simulink library "xrbsComm_r3"  (Simulink 5.1)
libraries: xbsIndex_r3 x775, xrbsComm_r3 x1
(part 3 of 6)

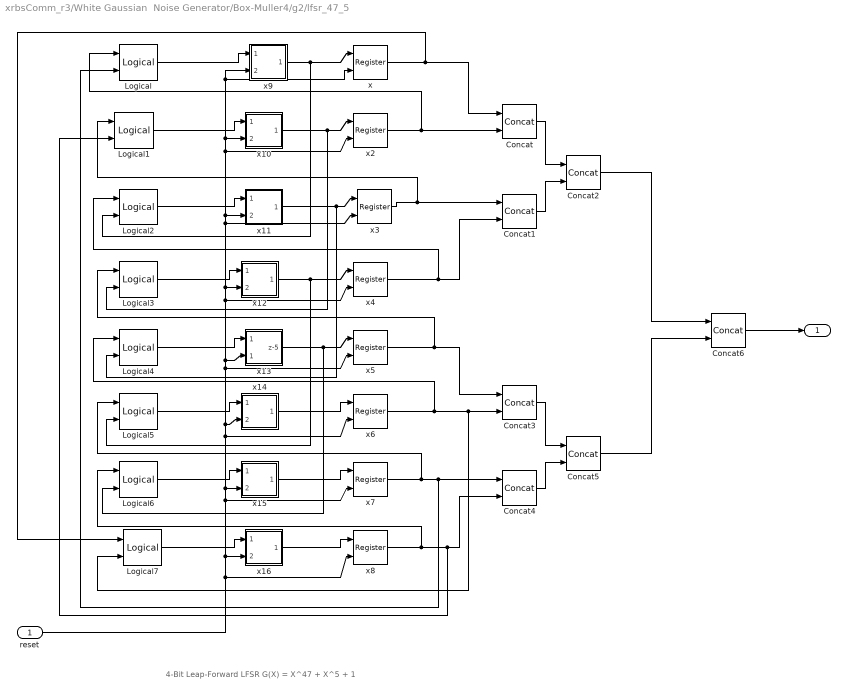
== system xrbsComm_r3/White Gaussian  Noise Generator/Box-Muller4/g2/lfsr_47_5 ==
  note: 4-Bit Leap-Forward LFSR G(X) = X^47 + X^5 + 1
  reset : Inport
  Concat{,1..6} (7 alike) : xbsIndex_r3/Concat  explicit_period=off  period=1  dbl_ovrd=off
  Logical{,1..7} (8 alike) : xbsIndex_r3/Logical  logical_function=XOR  inputs=2  precision=User Defined  arith_type=Unsigned  n_bits=1  bin_pt=0  align_bp=on  latency=0  explicit_period=on  period=-1  en=off  dbl_ovrd=off
      settings: xl_area=[0, 0, 0, 0, 0, 0, 0]
  x : xbsIndex_r3/Register  init=init(1)  reg_only_valid=off  explicit_period=off  period=1  rst=on  en=off  out_en=off  dbl_ovrd=off
      settings: xl_area=[0, 0, 0, 0, 0, 0, 0]
  x10 : Subsystem  mask{init=init(10:8:42)}
  x11 : Subsystem  mask{init=init(11:8:43)}
  x12 : Subsystem  mask{init=init(12:8:44)}
  x13 : Subsystem  mask{init=init(13:8:45)}
  x14 : Subsystem  mask{init=init(14:8:46)}
  x15 : Subsystem  mask{init=init(15:8:47)}
  x16 : Subsystem  mask{init=init(16:8:40)}
  x2 : xbsIndex_r3/Register  init=init(2)  reg_only_valid=off  explicit_period=off  period=1  rst=on  en=off  out_en=off  dbl_ovrd=off
      settings: xl_area=[0, 0, 0, 0, 0, 0, 0]
  x3 : xbsIndex_r3/Register  init=init(3)  reg_only_valid=off  explicit_period=off  period=1  rst=on  en=off  out_en=off  dbl_ovrd=off
      settings: xl_area=[0, 0, 0, 0, 0, 0, 0]
  x4 : xbsIndex_r3/Register  init=init(4)  reg_only_valid=off  explicit_period=off  period=1  rst=on  en=off  out_en=off  dbl_ovrd=off
      settings: xl_area=[0, 0, 0, 0, 0, 0, 0]
  x5 : xbsIndex_r3/Register  init=init(5)  reg_only_valid=off  explicit_period=off  period=1  rst=on  en=off  out_en=off  dbl_ovrd=off
      settings: xl_area=[0, 0, 0, 0, 0, 0, 0]
  x6 : xbsIndex_r3/Register  init=init(6)  reg_only_valid=off  explicit_period=off  period=1  rst=on  en=off  out_en=off  dbl_ovrd=off
      settings: xl_area=[0, 0, 0, 0, 0, 0, 0]
  x7 : xbsIndex_r3/Register  init=init(7)  reg_only_valid=off  explicit_period=off  period=1  rst=on  en=off  out_en=off  dbl_ovrd=off
      settings: xl_area=[0, 0, 0, 0, 0, 0, 0]
  x8 : xbsIndex_r3/Register  init=init(8)  reg_only_valid=off  explicit_period=off  period=1  rst=on  en=off  out_en=off  dbl_ovrd=off
      settings: xl_area=[0, 0, 0, 0, 0, 0, 0]
  x9 : Subsystem  mask{init=init(9:8:41)}
  " " : Outport
  wires:
  Logical/1 -> x9/1(" ")
  x9/1(z-5) -> x/1, Logical2/2
  x/1 -> Concat/1, Logical7/1
  x2/1 -> Concat/2, Logical/1
  Concat/1 -> Concat2/1
  x3/1 -> Concat1/1, Logical1/1
  x4/1 -> Concat1/2, Logical2/1
  Concat1/1 -> Concat2/2
  Logical1/1 -> x10/1("  ")
  x10/1(z-5) -> x2/1, Logical3/2
  Logical2/1 -> x11/1(" ")
  x11/1(z-5) -> x3/1, Logical4/2
  Logical3/1 -> x12/1(" ")
  x12/1(z-5) -> x4/1, Logical5/2
  Logical4/1 -> x13/1(" ")
  x13/1(z-5) -> x5/1, Logical6/2
  Logical5/1 -> x14/1(" ")
  x14/1(z-5) -> x6/1
  Logical6/1 -> x15/1(" ")
  x15/1(z-5) -> x7/1
  Logical7/1 -> x16/1(" ")
  x16/1(z-4) -> x8/1
  x6/1 -> Logical4/1, Concat3/2, Logical7/2
  Concat3/1 -> Concat5/1
  Concat4/1 -> Concat5/2
  x5/1 -> Concat3/1, Logical3/1
  x7/1 -> Concat4/1, Logical/2, Logical5/1
  x8/1 -> Concat4/2, Logical1/2, Logical6/1
  Concat2/1 -> Concat6/1
  Concat5/1 -> Concat6/2
  Concat6/1 -> " "/1
  reset/1 -> x9/2(reset), x/2, x10/2(reset), x2/2, x11/2(reset), x3/2, x12/2(reset), x4/2, x13/2(" 1"), x5/2, x14/2(reset), x6/2, x15/2(reset), x7/2, x16/2(reset), x8/2

== system xrbsComm_r3/White Gaussian  Noise Generator/Box-Muller1/f/lfsr_17_2/x1 ==
  " " : Inport
  " reset" : Inport  Port=2
  ASR : Subsystem  mask{init=[init(1) init(2)]}
      mask prompts: init "Initial Value"
      mask init:
      | init_size = size(init);
      | asr_length = init_size(2);
  Register4 : xbsIndex_r3/Register  init=init(3)  reg_only_valid=off  explicit_period=on  period=-1  rst=on  en=off  out_en=off  dbl_ovrd=off
      settings: xl_area=[0, 0, 0, 0, 0, 0, 0]
  z-3 : Outport
  wires:
  " "/1 -> Register4/1
  ASR/1(dout) -> z-3/1
  Register4/1 -> ASR/1(din)
  " reset"/1 -> Register4/2

== system xrbsComm_r3/White Gaussian  Noise Generator/Box-Muller1/f/lfsr_17_2/x5 ==
  " " : Inport
  reset : Inport  Port=2
  ASR : Subsystem  mask{init=[init(1) init(2) init(3)]}
      mask prompts: init "Initial Value"
      mask init:
      | init_size = size(init);
      | asr_length = init_size(2);
  Register5 : xbsIndex_r3/Register  init=init(4)  reg_only_valid=off  explicit_period=on  period=-1  rst=on  en=off  out_en=off  dbl_ovrd=off
      settings: xl_area=[0, 0, 0, 0, 0, 0, 0]
  z-4 : Outport
  wires:
  ASR/1(dout) -> z-4/1
  Register5/1 -> ASR/1(din)
  " "/1 -> Register5/1
  reset/1 -> Register5/2

== system xrbsComm_r3/White Gaussian  Noise Generator/Box-Muller1/f/lfsr_17_2/x6 ==
  " " : Inport
  " reset" : Inport  Port=2
  ASR : Subsystem  mask{init=[init(2) init(1)]}
      mask prompts: init "Initial Value"
      mask init:
      | init_size = size(init);
      | asr_length = init_size(2);
  Register4 : xbsIndex_r3/Register  init=init(3)  reg_only_valid=off  explicit_period=on  period=-1  rst=on  en=off  out_en=off  dbl_ovrd=off
      settings: xl_area=[0, 0, 0, 0, 0, 0, 0]
  z-3 : Outport
  wires:
  ASR/1(dout) -> z-3/1
  " "/1 -> Register4/1
  Register4/1 -> ASR/1(din)
  " reset"/1 -> Register4/2

== system xrbsComm_r3/White Gaussian  Noise Generator/Box-Muller1/f/lfsr_17_2/x7 ==
  " " : Inport
  reset : Inport  Port=2
  ASR : Subsystem  mask{init=[init(2) init(1)]}
      mask prompts: init "Initial Value"
      mask init:
      | init_size = size(init);
      | asr_length = init_size(2);
  Register4 : xbsIndex_r3/Register  init=init(3)  reg_only_valid=off  explicit_period=on  period=-1  rst=on  en=off  out_en=off  dbl_ovrd=off
      settings: xl_area=[0, 0, 0, 0, 0, 0, 0]
  z-3 : Outport
  wires:
  " "/1 -> Register4/1
  ASR/1(dout) -> z-3/1
  Register4/1 -> ASR/1(din)
  reset/1 -> Register4/2

== system xrbsComm_r3/White Gaussian  Noise Generator/Box-Muller1/f/lfsr_25_1/x1 ==
  " " : Inport
  reset : Inport  Port=2
  ASR : Subsystem  mask{init=[init(4) init(3) init(2) init(1)]}
      mask prompts: init "Initial Value"
      mask init:
      | init_size = size(init);
      | asr_length = init_size(2);
  Register : xbsIndex_r3/Register  init=init(5)  reg_only_valid=off  explicit_period=on  period=-1  rst=on  en=off  out_en=off  dbl_ovrd=off
      settings: xl_area=[0, 0, 0, 0, 0, 0, 0]
  z-5 : Outport
  wires:
  Register/1 -> ASR/1(din)
  ASR/1(dout) -> z-5/1
  " "/1 -> Register/1
  reset/1 -> Register/2

== system xrbsComm_r3/White Gaussian  Noise Generator/Box-Muller1/f/lfsr_25_1/x5 ==
  " " : Inport
  reset : Inport  Port=2
  ASR : Subsystem  mask{init=[init(5) init(4) init(3) init(2) init(1)]}
      mask prompts: init "Initial Value"
      mask init:
      | init_size = size(init);
      | asr_length = init_size(2);
  Register : xbsIndex_r3/Register  init=init(6)  reg_only_valid=off  explicit_period=on  period=-1  rst=on  en=off  out_en=off  dbl_ovrd=off
      settings: xl_area=[0, 0, 0, 0, 0, 0, 0]
  z-6 : Outport
  wires:
  Register/1 -> ASR/1(din)
  ASR/1(dout) -> z-6/1
  " "/1 -> Register/1
  reset/1 -> Register/2

== system xrbsComm_r3/White Gaussian  Noise Generator/Box-Muller1/f/lfsr_25_1/x6 ==
  " " : Inport
  reset : Inport  Port=2
  ASR : Subsystem  mask{init=[init(4) init(3) init(2) init(1)]}
      mask prompts: init "Initial Value"
      mask init:
      | init_size = size(init);
      | asr_length = init_size(2);
  Register : xbsIndex_r3/Register  init=init(5)  reg_only_valid=off  explicit_period=on  period=-1  rst=on  en=off  out_en=off  dbl_ovrd=off
      settings: xl_area=[0, 0, 0, 0, 0, 0, 0]
  z-5 : Outport
  wires:
  Register/1 -> ASR/1(din)
  ASR/1(dout) -> z-5/1
  " "/1 -> Register/1
  reset/1 -> Register/2

== system xrbsComm_r3/White Gaussian  Noise Generator/Box-Muller1/f/lfsr_25_1/x7 ==
  " " : Inport
  reset : Inport  Port=2
  ASR : Subsystem  mask{init=[init(4) init(3) init(2) init(1)]}
      mask prompts: init "Initial Value"
      mask init:
      | init_size = size(init);
      | asr_length = init_size(2);
  Register : xbsIndex_r3/Register  init=init(5)  reg_only_valid=off  explicit_period=on  period=-1  rst=on  en=off  out_en=off  dbl_ovrd=off
      settings: xl_area=[0, 0, 0, 0, 0, 0, 0]
  z-5 : Outport
  wires:
  Register/1 -> ASR/1(din)
  ASR/1(dout) -> z-5/1
  " "/1 -> Register/1
  reset/1 -> Register/2

== system xrbsComm_r3/White Gaussian  Noise Generator/Box-Muller1/f/lfsr_29_2/x5 ==
  " " : Inport
  reset : Inport  Port=2
  ASR : Subsystem  mask{init=[init(6) init(5) init(4) init(3) init(2) init(1)]}
      mask prompts: init "Initial Value"
      mask init:
      | init_size = size(init);
      | asr_length = init_size(2);
  Register : xbsIndex_r3/Register  init=init(7)  reg_only_valid=off  explicit_period=on  period=-1  rst=on  en=off  out_en=off  dbl_ovrd=off
      settings: xl_area=[0, 0, 0, 0, 0, 0, 0]
  z-7 : Outport
  wires:
  ASR/1(dout) -> z-7/1
  Register/1 -> ASR/1(din)
  " "/1 -> Register/1
  reset/1 -> Register/2

== system xrbsComm_r3/White Gaussian  Noise Generator/Box-Muller1/f/lfsr_29_2/x6 ==
  " " : Inport
  reset : Inport  Port=2
  ASR : Subsystem  mask{init=[init(5) init(4) init(3) init(2) init(1)]}
      mask prompts: init "Initial Value"
      mask init:
      | init_size = size(init);
      | asr_length = init_size(2);
  Register : xbsIndex_r3/Register  init=init(6)  reg_only_valid=off  explicit_period=on  period=-1  rst=on  en=off  out_en=off  dbl_ovrd=off
      settings: xl_area=[0, 0, 0, 0, 0, 0, 0]
  z-6 : Outport
  wires:
  ASR/1(dout) -> z-6/1
  Register/1 -> ASR/1(din)
  " "/1 -> Register/1
  reset/1 -> Register/2

== system xrbsComm_r3/White Gaussian  Noise Generator/Box-Muller1/f/lfsr_29_2/x7 ==
  " " : Inport
  reset : Inport  Port=2
  ASR : Subsystem  mask{init=[init(5) init(4) init(3) init(2) init(1)]}
      mask prompts: init "Initial Value"
      mask init:
      | init_size = size(init);
      | asr_length = init_size(2);
  Register : xbsIndex_r3/Register  init=init(6)  reg_only_valid=off  explicit_period=on  period=-1  rst=on  en=off  out_en=off  dbl_ovrd=off
      settings: xl_area=[0, 0, 0, 0, 0, 0, 0]
  z-6 : Outport
  wires:
  ASR/1(dout) -> z-6/1
  Register/1 -> ASR/1(din)
  " "/1 -> Register/1
  reset/1 -> Register/2

== system xrbsComm_r3/White Gaussian  Noise Generator/Box-Muller1/f/lfsr_29_2/x8 ==
  " " : Inport
  reset : Inport  Port=2
  ASR : Subsystem  mask{init=[init(5) init(4) init(3) init(2) init(1)]}
      mask prompts: init "Initial Value"
      mask init:
      | init_size = size(init);
      | asr_length = init_size(2);
  Register : xbsIndex_r3/Register  init=init(6)  reg_only_valid=off  explicit_period=on  period=-1  rst=on  en=off  out_en=off  dbl_ovrd=off
      settings: xl_area=[0, 0, 0, 0, 0, 0, 0]
  z-6 : Outport
  wires:
  ASR/1(dout) -> z-6/1
  Register/1 -> ASR/1(din)
  " "/1 -> Register/1
  reset/1 -> Register/2

== system xrbsComm_r3/White Gaussian  Noise Generator/Box-Muller1/f/lfsr_31_2/x5 ==
  " " : Inport
  reset : Inport  Port=2
  ASR : Subsystem  mask{init=[init(6) init(5) init(4) init(3) init(2) init(1)]}
      mask prompts: init "Initial Value"
      mask init:
      | init_size = size(init);
      | asr_length = init_size(2);
  Register : xbsIndex_r3/Register  init=init(7)  reg_only_valid=off  explicit_period=on  period=-1  rst=on  en=off  out_en=off  dbl_ovrd=off
      settings: xl_area=[0, 0, 0, 0, 0, 0, 0]
  z-7 : Outport
  wires:
  Register/1 -> ASR/1(din)
  ASR/1(dout) -> z-7/1
  " "/1 -> Register/1
  reset/1 -> Register/2

== system xrbsComm_r3/White Gaussian  Noise Generator/Box-Muller1/f/lfsr_31_2/x6 ==
  " " : Inport
  reset : Inport  Port=2
  ASR : Subsystem  mask{init=[init(6) init(5) init(4) init(3) init(2) init(1)]}
      mask prompts: init "Initial Value"
      mask init:
      | init_size = size(init);
      | asr_length = init_size(2);
  Register : xbsIndex_r3/Register  init=init(7)  reg_only_valid=off  explicit_period=on  period=-1  rst=on  en=off  out_en=off  dbl_ovrd=off
      settings: xl_area=[0, 0, 0, 0, 0, 0, 0]
  z-7 : Outport
  wires:
  Register/1 -> ASR/1(din)
  " "/1 -> Register/1
  ASR/1(dout) -> z-7/1
  reset/1 -> Register/2

== system xrbsComm_r3/White Gaussian  Noise Generator/Box-Muller1/f/lfsr_31_2/x7 ==
  " " : Inport
  reset : Inport  Port=2
  ASR : Subsystem  mask{init=[init(6) init(5) init(4) init(3) init(2) init(1)]}
      mask prompts: init "Initial Value"
      mask init:
      | init_size = size(init);
      | asr_length = init_size(2);
  Register : xbsIndex_r3/Register  init=init(7)  reg_only_valid=off  explicit_period=on  period=-1  rst=on  en=off  out_en=off  dbl_ovrd=off
      settings: xl_area=[0, 0, 0, 0, 0, 0, 0]
  z-7 : Outport
  wires:
  Register/1 -> ASR/1(din)
  ASR/1(dout) -> z-7/1
  " "/1 -> Register/1
  reset/1 -> Register/2

== system xrbsComm_r3/White Gaussian  Noise Generator/Box-Muller1/f/lfsr_31_2/x8 ==
  " " : Inport
  reset : Inport  Port=2
  ASR : Subsystem  mask{init=[init(5) init(4) init(3) init(2) init(1)]}
      mask prompts: init "Initial Value"
      mask init:
      | init_size = size(init);
      | asr_length = init_size(2);
  Register : xbsIndex_r3/Register  init=init(6)  reg_only_valid=off  explicit_period=on  period=-1  rst=on  en=off  out_en=off  dbl_ovrd=off
      settings: xl_area=[0, 0, 0, 0, 0, 0, 0]
  z-6 : Outport
  wires:
  Register/1 -> ASR/1(din)
  " "/1 -> Register/1
  ASR/1(dout) -> z-6/1
  reset/1 -> Register/2

== system xrbsComm_r3/White Gaussian  Noise Generator/Box-Muller1/f/lfsr_41_2/x1 ==
  " " : Inport
  reset : Inport  Port=2
  ASR : Subsystem  mask{init=[init(8) init(7) init(6) init(5) init(4) init(3) init(2) init(1)]}
      mask prompts: init "Initial Value"
      mask init:
      | init_size = size(init);
      | asr_length = init_size(2);
  Register1 : xbsIndex_r3/Register  init=init(9)  reg_only_valid=off  explicit_period=on  period=-1  rst=on  en=off  out_en=off  dbl_ovrd=off
      settings: xl_area=[0, 0, 0, 0, 0, 0, 0]
  z-9 : Outport
  wires:
  ASR/1(dout) -> z-9/1
  " "/1 -> Register1/1
  Register1/1 -> ASR/1(din)
  reset/1 -> Register1/2

== system xrbsComm_r3/White Gaussian  Noise Generator/Box-Muller1/f/lfsr_41_2/x5 ==
  " " : Inport
  reset : Inport  Port=2
  ASR : Subsystem  mask{init=[init(9) init(8) init(7) init(6) init(5) init(4) init(3) init(2) init(1)]}
      mask prompts: init "Initial Value"
      mask init:
      | init_size = size(init);
      | asr_length = init_size(2);
  Register : xbsIndex_r3/Register  init=init(10)  reg_only_valid=off  explicit_period=on  period=-1  rst=on  en=off  out_en=off  dbl_ovrd=off
      settings: xl_area=[0, 0, 0, 0, 0, 0, 0]
  z-10 : Outport
  wires:
  Register/1 -> ASR/1(din)
  ASR/1(dout) -> z-10/1
  " "/1 -> Register/1
  reset/1 -> Register/2

== system xrbsComm_r3/White Gaussian  Noise Generator/Box-Muller1/f/lfsr_41_2/x6 ==
  " " : Inport
  reset : Inport  Port=2
  ASR : Subsystem  mask{init=[init(8) init(7) init(6) init(5) init(4) init(3) init(2) init(1)]}
      mask prompts: init "Initial Value"
      mask init:
      | init_size = size(init);
      | asr_length = init_size(2);
  Register1 : xbsIndex_r3/Register  init=init(9)  reg_only_valid=off  explicit_period=on  period=-1  rst=on  en=off  out_en=off  dbl_ovrd=off
      settings: xl_area=[0, 0, 0, 0, 0, 0, 0]
  z-9 : Outport
  wires:
  ASR/1(dout) -> z-9/1
  " "/1 -> Register1/1
  Register1/1 -> ASR/1(din)
  reset/1 -> Register1/2

== system xrbsComm_r3/White Gaussian  Noise Generator/Box-Muller1/f/lfsr_41_2/x7 ==
  " " : Inport
  reset : Inport  Port=2
  ASR : Subsystem  mask{init=[init(8) init(7) init(6) init(5) init(4) init(3) init(2) init(1)]}
      mask prompts: init "Initial Value"
      mask init:
      | init_size = size(init);
      | asr_length = init_size(2);
  Register1 : xbsIndex_r3/Register  init=init(9)  reg_only_valid=off  explicit_period=on  period=-1  rst=on  en=off  out_en=off  dbl_ovrd=off
      settings: xl_area=[0, 0, 0, 0, 0, 0, 0]
  z-9 : Outport
  wires:
  ASR/1(dout) -> z-9/1
  Register1/1 -> ASR/1(din)
  " "/1 -> Register1/1
  reset/1 -> Register1/2

== system xrbsComm_r3/White Gaussian  Noise Generator/Box-Muller1/g/lfsr_47_5/x10 ==
  "  " : Inport
  reset : Inport  Port=2
  ASR : Subsystem  mask{init=[init(4) init(3) init(2) init(1)]}
      mask prompts: init "Initial Value"
      mask init:
      | init_size = size(init);
      | asr_length = init_size(2);
  Register5 : xbsIndex_r3/Register  init=init(5)  reg_only_valid=off  explicit_period=on  period=-1  rst=on  en=off  out_en=off  dbl_ovrd=off
      settings: xl_area=[0, 0, 0, 0, 0, 0, 0]
  z-5 : Outport
  wires:
  ASR/1(dout) -> z-5/1
  Register5/1 -> ASR/1(din)
  "  "/1 -> Register5/1
  reset/1 -> Register5/2

== system xrbsComm_r3/White Gaussian  Noise Generator/Box-Muller1/g/lfsr_47_5/x11 ==
  " " : Inport
  reset : Inport  Port=2
  ASR : Subsystem  mask{init=[init(4) init(3) init(2) init(1)]}
      mask prompts: init "Initial Value"
      mask init:
      | init_size = size(init);
      | asr_length = init_size(2);
  Register : xbsIndex_r3/Register  init=init(5)  reg_only_valid=off  explicit_period=on  period=-1  rst=on  en=off  out_en=off  dbl_ovrd=off
      settings: xl_area=[0, 0, 0, 0, 0, 0, 0]
  z-5 : Outport
  wires:
  ASR/1(dout) -> z-5/1
  Register/1 -> ASR/1(din)
  " "/1 -> Register/1
  reset/1 -> Register/2

== system xrbsComm_r3/White Gaussian  Noise Generator/Box-Muller1/g/lfsr_47_5/x12 ==
  " " : Inport
  reset : Inport  Port=2
  ASR : Subsystem  mask{init=[init(4) init(3) init(2) init(1)]}
      mask prompts: init "Initial Value"
      mask init:
      | init_size = size(init);
      | asr_length = init_size(2);
  Register : xbsIndex_r3/Register  init=init(5)  reg_only_valid=off  explicit_period=on  period=-1  rst=on  en=off  out_en=off  dbl_ovrd=off
      settings: xl_area=[0, 0, 0, 0, 0, 0, 0]
  z-5 : Outport
  wires:
  ASR/1(dout) -> z-5/1
  Register/1 -> ASR/1(din)
  " "/1 -> Register/1
  reset/1 -> Register/2

== system xrbsComm_r3/White Gaussian  Noise Generator/Box-Muller1/g/lfsr_47_5/x13 ==
  note: reset
  " " : Inport
  " 1" : Inport  Port=2
  ASR : Subsystem  mask{init=[init(4) init(3) init(2) init(1)]}
      mask prompts: init "Initial Value"
      mask init:
      | init_size = size(init);
      | asr_length = init_size(2);
  Register : xbsIndex_r3/Register  init=init(5)  reg_only_valid=off  explicit_period=on  period=-1  rst=on  en=off  out_en=off  dbl_ovrd=off
      settings: xl_area=[0, 0, 0, 0, 0, 0, 0]
  z-5 : Outport
  wires:
  ASR/1(dout) -> z-5/1
  Register/1 -> ASR/1(din)
  " "/1 -> Register/1
  " 1"/1 -> Register/2

== system xrbsComm_r3/White Gaussian  Noise Generator/Box-Muller1/g/lfsr_47_5/x14 ==
  " " : Inport
  reset : Inport  Port=2
  ASR : Subsystem  mask{init=[init(4) init(3) init(2) init(1)]}
      mask prompts: init "Initial Value"
      mask init:
      | init_size = size(init);
      | asr_length = init_size(2);
  Register : xbsIndex_r3/Register  init=init(5)  reg_only_valid=off  explicit_period=on  period=-1  rst=on  en=off  out_en=off  dbl_ovrd=off
      settings: xl_area=[0, 0, 0, 0, 0, 0, 0]
  z-5 : Outport
  wires:
  ASR/1(dout) -> z-5/1
  Register/1 -> ASR/1(din)
  " "/1 -> Register/1
  reset/1 -> Register/2

== system xrbsComm_r3/White Gaussian  Noise Generator/Box-Muller1/g/lfsr_47_5/x15 ==
  " " : Inport
  reset : Inport  Port=2
  ASR : Subsystem  mask{init=[init(4) init(3) init(2) init(1)]}
      mask prompts: init "Initial Value"
      mask init:
      | init_size = size(init);
      | asr_length = init_size(2);
  Register : xbsIndex_r3/Register  init=init(5)  reg_only_valid=off  explicit_period=on  period=-1  rst=on  en=off  out_en=off  dbl_ovrd=off
      settings: xl_area=[0, 0, 0, 0, 0, 0, 0]
  z-5 : Outport
  wires:
  ASR/1(dout) -> z-5/1
  Register/1 -> ASR/1(din)
  " "/1 -> Register/1
  reset/1 -> Register/2

== system xrbsComm_r3/White Gaussian  Noise Generator/Box-Muller1/g/lfsr_47_5/x16 ==
  " " : Inport
  reset : Inport  Port=2
  ASR : Subsystem  mask{init=[init(3) init(2) init(1)]}
      mask prompts: init "Initial Value"
      mask init:
      | init_size = size(init);
      | asr_length = init_size(2);
  Register : xbsIndex_r3/Register  init=init(4)  reg_only_valid=off  explicit_period=on  period=-1  rst=on  en=off  out_en=off  dbl_ovrd=off
      settings: xl_area=[0, 0, 0, 0, 0, 0, 0]
  z-4 : Outport
  wires:
  ASR/1(dout) -> z-4/1
  Register/1 -> ASR/1(din)
  " "/1 -> Register/1
  reset/1 -> Register/2

== system xrbsComm_r3/White Gaussian  Noise Generator/Box-Muller1/g/lfsr_47_5/x9 ==
  " " : Inport
  reset : Inport  Port=2
  ASR : Subsystem  mask{init=[init(4) init(3) init(2) init(1)]}
      mask prompts: init "Initial Value"
      mask init:
      | init_size = size(init);
      | asr_length = init_size(2);
  Register : xbsIndex_r3/Register  init=init(5)  reg_only_valid=off  explicit_period=on  period=-1  rst=on  en=off  out_en=off  dbl_ovrd=off
      settings: xl_area=[0, 0, 0, 0, 0, 0, 0]
  z-5 : Outport
  wires:
  ASR/1(dout) -> z-5/1
  Register/1 -> ASR/1(din)
  " "/1 -> Register/1
  reset/1 -> Register/2

== system xrbsComm_r3/White Gaussian  Noise Generator/Box-Muller2/fr1/lfsr_17_2/x1 ==
  " " : Inport
  " reset" : Inport  Port=2
  ASR : Subsystem  mask{init=[init(2) init(1)]}
      mask prompts: init "Initial Value"
      mask init:
      | init_size = size(init);
      | asr_length = init_size(2);
  Register4 : xbsIndex_r3/Register  init=init(3)  reg_only_valid=off  explicit_period=on  period=-1  rst=on  en=off  out_en=off  dbl_ovrd=off
      settings: xl_area=[0, 0, 0, 0, 0, 0, 0]
  z-3 : Outport
  wires:
  " "/1 -> Register4/1
  ASR/1(dout) -> z-3/1
  Register4/1 -> ASR/1(din)
  " reset"/1 -> Register4/2

== system xrbsComm_r3/White Gaussian  Noise Generator/Box-Muller2/fr1/lfsr_17_2/x5 ==
  " " : Inport
  reset : Inport  Port=2
  ASR : Subsystem  mask{init=[init(3) init(2) init(1)]}
      mask prompts: init "Initial Value"
      mask init:
      | init_size = size(init);
      | asr_length = init_size(2);
  Register5 : xbsIndex_r3/Register  init=init(4)  reg_only_valid=off  explicit_period=on  period=-1  rst=on  en=off  out_en=off  dbl_ovrd=off
      settings: xl_area=[0, 0, 0, 0, 0, 0, 0]
  z-4 : Outport
  wires:
  ASR/1(dout) -> z-4/1
  Register5/1 -> ASR/1(din)
  " "/1 -> Register5/1
  reset/1 -> Register5/2

== system xrbsComm_r3/White Gaussian  Noise Generator/Box-Muller2/fr1/lfsr_17_2/x6 ==
  " " : Inport
  " reset" : Inport  Port=2
  ASR : Subsystem  mask{init=[init(2) init(1)]}
      mask prompts: init "Initial Value"
      mask init:
      | init_size = size(init);
      | asr_length = init_size(2);
  Register4 : xbsIndex_r3/Register  init=init(3)  reg_only_valid=off  explicit_period=on  period=-1  rst=on  en=off  out_en=off  dbl_ovrd=off
      settings: xl_area=[0, 0, 0, 0, 0, 0, 0]
  z-3 : Outport
  wires:
  ASR/1(dout) -> z-3/1
  " "/1 -> Register4/1
  Register4/1 -> ASR/1(din)
  " reset"/1 -> Register4/2

== system xrbsComm_r3/White Gaussian  Noise Generator/Box-Muller2/fr1/lfsr_17_2/x7 ==
  " " : Inport
  reset : Inport  Port=2
  ASR : Subsystem  mask{init=[init(2) init(1)]}
      mask prompts: init "Initial Value"
      mask init:
      | init_size = size(init);
      | asr_length = init_size(2);
  Register4 : xbsIndex_r3/Register  init=init(3)  reg_only_valid=off  explicit_period=on  period=-1  rst=on  en=off  out_en=off  dbl_ovrd=off
      settings: xl_area=[0, 0, 0, 0, 0, 0, 0]
  z-3 : Outport
  wires:
  " "/1 -> Register4/1
  ASR/1(dout) -> z-3/1
  Register4/1 -> ASR/1(din)
  reset/1 -> Register4/2

== system xrbsComm_r3/White Gaussian  Noise Generator/Box-Muller2/fr1/lfsr_25_2/x1 ==
  " " : Inport
  reset : Inport  Port=2
  ASR : Subsystem  mask{init=[init(4) init(3) init(2) init(1)]}
      mask prompts: init "Initial Value"
      mask init:
      | init_size = size(init);
      | asr_length = init_size(2);
  Register : xbsIndex_r3/Register  init=init(5)  reg_only_valid=off  explicit_period=on  period=-1  rst=on  en=off  out_en=off  dbl_ovrd=off
      settings: xl_area=[0, 0, 0, 0, 0, 0, 0]
  z-5 : Outport
  wires:
  Register/1 -> ASR/1(din)
  ASR/1(dout) -> z-5/1
  " "/1 -> Register/1
  reset/1 -> Register/2

== system xrbsComm_r3/White Gaussian  Noise Generator/Box-Muller2/fr1/lfsr_25_2/x5 ==
  " " : Inport
  reset : Inport  Port=2
  ASR : Subsystem  mask{init=[init(5) init(4) init(3) init(2) init(1)]}
      mask prompts: init "Initial Value"
      mask init:
      | init_size = size(init);
      | asr_length = init_size(2);
  Register : xbsIndex_r3/Register  init=init(6)  reg_only_valid=off  explicit_period=on  period=-1  rst=on  en=off  out_en=off  dbl_ovrd=off
      settings: xl_area=[0, 0, 0, 0, 0, 0, 0]
  z-6 : Outport
  wires:
  Register/1 -> ASR/1(din)
  ASR/1(dout) -> z-6/1
  " "/1 -> Register/1
  reset/1 -> Register/2

== system xrbsComm_r3/White Gaussian  Noise Generator/Box-Muller2/fr1/lfsr_25_2/x6 ==
  " " : Inport
  reset : Inport  Port=2
  ASR : Subsystem  mask{init=[init(4) init(3) init(2) init(1)]}
      mask prompts: init "Initial Value"
      mask init:
      | init_size = size(init);
      | asr_length = init_size(2);
  Register : xbsIndex_r3/Register  init=init(5)  reg_only_valid=off  explicit_period=on  period=-1  rst=on  en=off  out_en=off  dbl_ovrd=off
      settings: xl_area=[0, 0, 0, 0, 0, 0, 0]
  z-5 : Outport
  wires:
  Register/1 -> ASR/1(din)
  ASR/1(dout) -> z-5/1
  " "/1 -> Register/1
  reset/1 -> Register/2

== system xrbsComm_r3/White Gaussian  Noise Generator/Box-Muller2/fr1/lfsr_25_2/x7 ==
  " " : Inport
  reset : Inport  Port=2
  ASR : Subsystem  mask{init=[init(4) init(3) init(2) init(1)]}
      mask prompts: init "Initial Value"
      mask init:
      | init_size = size(init);
      | asr_length = init_size(2);
  Register : xbsIndex_r3/Register  init=init(5)  reg_only_valid=off  explicit_period=on  period=-1  rst=on  en=off  out_en=off  dbl_ovrd=off
      settings: xl_area=[0, 0, 0, 0, 0, 0, 0]
  z-5 : Outport
  wires:
  Register/1 -> ASR/1(din)
  ASR/1(dout) -> z-5/1
  " "/1 -> Register/1
  reset/1 -> Register/2

== system xrbsComm_r3/White Gaussian  Noise Generator/Box-Muller2/fr1/lfsr_29_2/x5 ==
  " " : Inport
  reset : Inport  Port=2
  ASR : Subsystem  mask{init=[init(6) init(5) init(4) init(3) init(2) init(1)]}
      mask prompts: init "Initial Value"
      mask init:
      | init_size = size(init);
      | asr_length = init_size(2);
  Register : xbsIndex_r3/Register  init=init(7)  reg_only_valid=off  explicit_period=on  period=-1  rst=on  en=off  out_en=off  dbl_ovrd=off
      settings: xl_area=[0, 0, 0, 0, 0, 0, 0]
  z-7 : Outport
  wires:
  ASR/1(dout) -> z-7/1
  Register/1 -> ASR/1(din)
  " "/1 -> Register/1
  reset/1 -> Register/2

== system xrbsComm_r3/White Gaussian  Noise Generator/Box-Muller2/fr1/lfsr_29_2/x6 ==
  " " : Inport
  reset : Inport  Port=2
  ASR : Subsystem  mask{init=[init(5) init(4) init(3) init(2) init(1)]}
      mask prompts: init "Initial Value"
      mask init:
      | init_size = size(init);
      | asr_length = init_size(2);
  Register : xbsIndex_r3/Register  init=init(6)  reg_only_valid=off  explicit_period=on  period=-1  rst=on  en=off  out_en=off  dbl_ovrd=off
      settings: xl_area=[0, 0, 0, 0, 0, 0, 0]
  z-6 : Outport
  wires:
  ASR/1(dout) -> z-6/1
  Register/1 -> ASR/1(din)
  " "/1 -> Register/1
  reset/1 -> Register/2

== system xrbsComm_r3/White Gaussian  Noise Generator/Box-Muller2/fr1/lfsr_29_2/x7 ==
  " " : Inport
  reset : Inport  Port=2
  ASR : Subsystem  mask{init=[init(5) init(4) init(3) init(2) init(1)]}
      mask prompts: init "Initial Value"
      mask init:
      | init_size = size(init);
      | asr_length = init_size(2);
  Register : xbsIndex_r3/Register  init=init(6)  reg_only_valid=off  explicit_period=on  period=-1  rst=on  en=off  out_en=off  dbl_ovrd=off
      settings: xl_area=[0, 0, 0, 0, 0, 0, 0]
  z-6 : Outport
  wires:
  ASR/1(dout) -> z-6/1
  Register/1 -> ASR/1(din)
  " "/1 -> Register/1
  reset/1 -> Register/2

== system xrbsComm_r3/White Gaussian  Noise Generator/Box-Muller2/fr1/lfsr_29_2/x8 ==
  " " : Inport
  reset : Inport  Port=2
  ASR : Subsystem  mask{init=[init(5) init(4) init(3) init(2) init(1)]}
      mask prompts: init "Initial Value"
      mask init:
      | init_size = size(init);
      | asr_length = init_size(2);
  Register : xbsIndex_r3/Register  init=init(6)  reg_only_valid=off  explicit_period=on  period=-1  rst=on  en=off  out_en=off  dbl_ovrd=off
      settings: xl_area=[0, 0, 0, 0, 0, 0, 0]
  z-6 : Outport
  wires:
  ASR/1(dout) -> z-6/1
  Register/1 -> ASR/1(din)
  " "/1 -> Register/1
  reset/1 -> Register/2

== system xrbsComm_r3/White Gaussian  Noise Generator/Box-Muller2/fr1/lfsr_31_2/x5 ==
  " " : Inport
  reset : Inport  Port=2
  ASR : Subsystem  mask{init=[init(6) init(5) init(4) init(3) init(2) init(1)]}
      mask prompts: init "Initial Value"
      mask init:
      | init_size = size(init);
      | asr_length = init_size(2);
  Register : xbsIndex_r3/Register  init=init(7)  reg_only_valid=off  explicit_period=on  period=-1  rst=on  en=off  out_en=off  dbl_ovrd=off
      settings: xl_area=[0, 0, 0, 0, 0, 0, 0]
  z-7 : Outport
  wires:
  Register/1 -> ASR/1(din)
  ASR/1(dout) -> z-7/1
  " "/1 -> Register/1
  reset/1 -> Register/2

== system xrbsComm_r3/White Gaussian  Noise Generator/Box-Muller2/fr1/lfsr_31_2/x6 ==
  " " : Inport
  reset : Inport  Port=2
  ASR : Subsystem  mask{init=[init(6) init(5) init(4) init(3) init(2) init(1)]}
      mask prompts: init "Initial Value"
      mask init:
      | init_size = size(init);
      | asr_length = init_size(2);
  Register : xbsIndex_r3/Register  init=init(7)  reg_only_valid=off  explicit_period=on  period=-1  rst=on  en=off  out_en=off  dbl_ovrd=off
      settings: xl_area=[0, 0, 0, 0, 0, 0, 0]
  z-7 : Outport
  wires:
  Register/1 -> ASR/1(din)
  " "/1 -> Register/1
  ASR/1(dout) -> z-7/1
  reset/1 -> Register/2

== system xrbsComm_r3/White Gaussian  Noise Generator/Box-Muller2/fr1/lfsr_31_2/x7 ==
  " " : Inport
  reset : Inport  Port=2
  ASR : Subsystem  mask{init=[init(6) init(5) init(4) init(3) init(2) init(1)]}
      mask prompts: init "Initial Value"
      mask init:
      | init_size = size(init);
      | asr_length = init_size(2);
  Register : xbsIndex_r3/Register  init=init(7)  reg_only_valid=off  explicit_period=on  period=-1  rst=on  en=off  out_en=off  dbl_ovrd=off
      settings: xl_area=[0, 0, 0, 0, 0, 0, 0]
  z-7 : Outport
  wires:
  Register/1 -> ASR/1(din)
  ASR/1(dout) -> z-7/1
  " "/1 -> Register/1
  reset/1 -> Register/2

== system xrbsComm_r3/White Gaussian  Noise Generator/Box-Muller2/fr1/lfsr_31_2/x8 ==
  " " : Inport
  reset : Inport  Port=2
  ASR : Subsystem  mask{init=[init(5) init(4) init(3) init(2) init(1)]}
      mask prompts: init "Initial Value"
      mask init:
      | init_size = size(init);
      | asr_length = init_size(2);
  Register : xbsIndex_r3/Register  init=init(6)  reg_only_valid=off  explicit_period=on  period=-1  rst=on  en=off  out_en=off  dbl_ovrd=off
      settings: xl_area=[0, 0, 0, 0, 0, 0, 0]
  z-6 : Outport
  wires:
  Register/1 -> ASR/1(din)
  " "/1 -> Register/1
  ASR/1(dout) -> z-6/1
  reset/1 -> Register/2

== system xrbsComm_r3/White Gaussian  Noise Generator/Box-Muller2/fr1/lfsr_41_2/x1 ==
  " " : Inport
  reset : Inport  Port=2
  ASR : Subsystem  mask{init=[init(8) init(7) init(6) init(5) init(4) init(3) init(2) init(1)]}
      mask prompts: init "Initial Value"
      mask init:
      | init_size = size(init);
      | asr_length = init_size(2);
  Register1 : xbsIndex_r3/Register  init=init(9)  reg_only_valid=off  explicit_period=on  period=-1  rst=on  en=off  out_en=off  dbl_ovrd=off
      settings: xl_area=[0, 0, 0, 0, 0, 0, 0]
  z-9 : Outport
  wires:
  ASR/1(dout) -> z-9/1
  " "/1 -> Register1/1
  Register1/1 -> ASR/1(din)
  reset/1 -> Register1/2

== system xrbsComm_r3/White Gaussian  Noise Generator/Box-Muller2/fr1/lfsr_41_2/x5 ==
  " " : Inport
  reset : Inport  Port=2
  ASR : Subsystem  mask{init=[init(9) init(8) init(7) init(6) init(5) init(4) init(3) init(2) init(1)]}
      mask prompts: init "Initial Value"
      mask init:
      | init_size = size(init);
      | asr_length = init_size(2);
  Register : xbsIndex_r3/Register  init=init(10)  reg_only_valid=off  explicit_period=on  period=-1  rst=on  en=off  out_en=off  dbl_ovrd=off
      settings: xl_area=[0, 0, 0, 0, 0, 0, 0]
  z-10 : Outport
  wires:
  Register/1 -> ASR/1(din)
  ASR/1(dout) -> z-10/1
  " "/1 -> Register/1
  reset/1 -> Register/2

== system xrbsComm_r3/White Gaussian  Noise Generator/Box-Muller2/fr1/lfsr_41_2/x6 ==
  " " : Inport
  reset : Inport  Port=2
  ASR : Subsystem  mask{init=[init(8) init(7) init(6) init(5) init(4) init(3) init(2) init(1)]}
      mask prompts: init "Initial Value"
      mask init:
      | init_size = size(init);
      | asr_length = init_size(2);
  Register1 : xbsIndex_r3/Register  init=init(9)  reg_only_valid=off  explicit_period=on  period=-1  rst=on  en=off  out_en=off  dbl_ovrd=off
      settings: xl_area=[0, 0, 0, 0, 0, 0, 0]
  z-9 : Outport
  wires:
  ASR/1(dout) -> z-9/1
  " "/1 -> Register1/1
  Register1/1 -> ASR/1(din)
  reset/1 -> Register1/2

== system xrbsComm_r3/White Gaussian  Noise Generator/Box-Muller2/fr1/lfsr_41_2/x7 ==
  " " : Inport
  reset : Inport  Port=2
  ASR : Subsystem  mask{init=[init(8) init(7) init(6) init(5) init(4) init(3) init(2) init(1)]}
      mask prompts: init "Initial Value"
      mask init:
      | init_size = size(init);
      | asr_length = init_size(2);
  Register1 : xbsIndex_r3/Register  init=init(9)  reg_only_valid=off  explicit_period=on  period=-1  rst=on  en=off  out_en=off  dbl_ovrd=off
      settings: xl_area=[0, 0, 0, 0, 0, 0, 0]
  z-9 : Outport
  wires:
  ASR/1(dout) -> z-9/1
  Register1/1 -> ASR/1(din)
  " "/1 -> Register1/1
  reset/1 -> Register1/2

== system xrbsComm_r3/White Gaussian  Noise Generator/Box-Muller2/g2/lfsr_47_5/x10 ==
  "  " : Inport
  reset : Inport  Port=2
  ASR : Subsystem  mask{init=[init(4) init(3) init(2) init(1)]}
      mask prompts: init "Initial Value"
      mask init:
      | init_size = size(init);
      | asr_length = init_size(2);
  Register5 : xbsIndex_r3/Register  init=init(5)  reg_only_valid=off  explicit_period=on  period=-1  rst=on  en=off  out_en=off  dbl_ovrd=off
      settings: xl_area=[0, 0, 0, 0, 0, 0, 0]
  z-5 : Outport
  wires:
  ASR/1(dout) -> z-5/1
  Register5/1 -> ASR/1(din)
  "  "/1 -> Register5/1
  reset/1 -> Register5/2

== system xrbsComm_r3/White Gaussian  Noise Generator/Box-Muller2/g2/lfsr_47_5/x11 ==
  " " : Inport
  reset : Inport  Port=2
  ASR : Subsystem  mask{init=[init(4) init(3) init(2) init(1)]}
      mask prompts: init "Initial Value"
      mask init:
      | init_size = size(init);
      | asr_length = init_size(2);
  Register : xbsIndex_r3/Register  init=init(5)  reg_only_valid=off  explicit_period=on  period=-1  rst=on  en=off  out_en=off  dbl_ovrd=off
      settings: xl_area=[0, 0, 0, 0, 0, 0, 0]
  z-5 : Outport
  wires:
  ASR/1(dout) -> z-5/1
  Register/1 -> ASR/1(din)
  " "/1 -> Register/1
  reset/1 -> Register/2

== system xrbsComm_r3/White Gaussian  Noise Generator/Box-Muller2/g2/lfsr_47_5/x12 ==
  " " : Inport
  reset : Inport  Port=2
  ASR : Subsystem  mask{init=[init(4) init(3) init(2) init(1)]}
      mask prompts: init "Initial Value"
      mask init:
      | init_size = size(init);
      | asr_length = init_size(2);
  Register : xbsIndex_r3/Register  init=init(5)  reg_only_valid=off  explicit_period=on  period=-1  rst=on  en=off  out_en=off  dbl_ovrd=off
      settings: xl_area=[0, 0, 0, 0, 0, 0, 0]
  z-5 : Outport
  wires:
  ASR/1(dout) -> z-5/1
  Register/1 -> ASR/1(din)
  " "/1 -> Register/1
  reset/1 -> Register/2

== system xrbsComm_r3/White Gaussian  Noise Generator/Box-Muller2/g2/lfsr_47_5/x13 ==
  note: reset
  " " : Inport
  " 1" : Inport  Port=2
  ASR : Subsystem  mask{init=[init(4) init(3) init(2) init(1)]}
      mask prompts: init "Initial Value"
      mask init:
      | init_size = size(init);
      | asr_length = init_size(2);
  Register : xbsIndex_r3/Register  init=init(5)  reg_only_valid=off  explicit_period=on  period=-1  rst=on  en=off  out_en=off  dbl_ovrd=off
      settings: xl_area=[0, 0, 0, 0, 0, 0, 0]
  z-5 : Outport
  wires:
  ASR/1(dout) -> z-5/1
  Register/1 -> ASR/1(din)
  " "/1 -> Register/1
  " 1"/1 -> Register/2

== system xrbsComm_r3/White Gaussian  Noise Generator/Box-Muller2/g2/lfsr_47_5/x14 ==
  " " : Inport
  reset : Inport  Port=2
  ASR : Subsystem  mask{init=[init(4) init(3) init(2) init(1)]}
      mask prompts: init "Initial Value"
      mask init:
      | init_size = size(init);
      | asr_length = init_size(2);
  Register : xbsIndex_r3/Register  init=init(5)  reg_only_valid=off  explicit_period=on  period=-1  rst=on  en=off  out_en=off  dbl_ovrd=off
      settings: xl_area=[0, 0, 0, 0, 0, 0, 0]
  z-5 : Outport
  wires:
  ASR/1(dout) -> z-5/1
  Register/1 -> ASR/1(din)
  " "/1 -> Register/1
  reset/1 -> Register/2

== system xrbsComm_r3/White Gaussian  Noise Generator/Box-Muller2/g2/lfsr_47_5/x15 ==
  " " : Inport
  reset : Inport  Port=2
  ASR : Subsystem  mask{init=[init(4) init(3) init(2) init(1)]}
      mask prompts: init "Initial Value"
      mask init:
      | init_size = size(init);
      | asr_length = init_size(2);
  Register : xbsIndex_r3/Register  init=init(5)  reg_only_valid=off  explicit_period=on  period=-1  rst=on  en=off  out_en=off  dbl_ovrd=off
      settings: xl_area=[0, 0, 0, 0, 0, 0, 0]
  z-5 : Outport
  wires:
  ASR/1(dout) -> z-5/1
  Register/1 -> ASR/1(din)
  " "/1 -> Register/1
  reset/1 -> Register/2

== system xrbsComm_r3/White Gaussian  Noise Generator/Box-Muller2/g2/lfsr_47_5/x16 ==
  " " : Inport
  reset : Inport  Port=2
  ASR : Subsystem  mask{init=[init(3) init(2) init(1)]}
      mask prompts: init "Initial Value"
      mask init:
      | init_size = size(init);
      | asr_length = init_size(2);
  Register : xbsIndex_r3/Register  init=init(4)  reg_only_valid=off  explicit_period=on  period=-1  rst=on  en=off  out_en=off  dbl_ovrd=off
      settings: xl_area=[0, 0, 0, 0, 0, 0, 0]
  z-4 : Outport
  wires:
  ASR/1(dout) -> z-4/1
  Register/1 -> ASR/1(din)
  " "/1 -> Register/1
  reset/1 -> Register/2

== system xrbsComm_r3/White Gaussian  Noise Generator/Box-Muller2/g2/lfsr_47_5/x9 ==
  " " : Inport
  reset : Inport  Port=2
  ASR : Subsystem  mask{init=[init(4) init(3) init(2) init(1)]}
      mask prompts: init "Initial Value"
      mask init:
      | init_size = size(init);
      | asr_length = init_size(2);
  Register : xbsIndex_r3/Register  init=init(5)  reg_only_valid=off  explicit_period=on  period=-1  rst=on  en=off  out_en=off  dbl_ovrd=off
      settings: xl_area=[0, 0, 0, 0, 0, 0, 0]
  z-5 : Outport
  wires:
  ASR/1(dout) -> z-5/1
  Register/1 -> ASR/1(din)
  " "/1 -> Register/1
  reset/1 -> Register/2

== system xrbsComm_r3/White Gaussian  Noise Generator/Box-Muller3/fr1/lfsr_17_2/x1 ==
  " " : Inport
  " reset" : Inport  Port=2
  ASR : Subsystem  mask{init=[init(2) init(1)]}
      mask prompts: init "Initial Value"
      mask init:
      | init_size = size(init);
      | asr_length = init_size(2);
  Register4 : xbsIndex_r3/Register  init=init(3)  reg_only_valid=off  explicit_period=on  period=-1  rst=on  en=off  out_en=off  dbl_ovrd=off
      settings: xl_area=[0, 0, 0, 0, 0, 0, 0]
  z-3 : Outport
  wires:
  " "/1 -> Register4/1
  ASR/1(dout) -> z-3/1
  Register4/1 -> ASR/1(din)
  " reset"/1 -> Register4/2

== system xrbsComm_r3/White Gaussian  Noise Generator/Box-Muller3/fr1/lfsr_17_2/x5 ==
  " " : Inport
  reset : Inport  Port=2
  ASR : Subsystem  mask{init=[init(3) init(2) init(1)]}
      mask prompts: init "Initial Value"
      mask init:
      | init_size = size(init);
      | asr_length = init_size(2);
  Register5 : xbsIndex_r3/Register  init=init(4)  reg_only_valid=off  explicit_period=on  period=-1  rst=on  en=off  out_en=off  dbl_ovrd=off
      settings: xl_area=[0, 0, 0, 0, 0, 0, 0]
  z-4 : Outport
  wires:
  ASR/1(dout) -> z-4/1
  Register5/1 -> ASR/1(din)
  " "/1 -> Register5/1
  reset/1 -> Register5/2

== system xrbsComm_r3/White Gaussian  Noise Generator/Box-Muller3/fr1/lfsr_17_2/x6 ==
  " " : Inport
  " reset" : Inport  Port=2
  ASR : Subsystem  mask{init=[init(2) init(1)]}
      mask prompts: init "Initial Value"
      mask init:
      | init_size = size(init);
      | asr_length = init_size(2);
  Register4 : xbsIndex_r3/Register  init=init(3)  reg_only_valid=off  explicit_period=on  period=-1  rst=on  en=off  out_en=off  dbl_ovrd=off
      settings: xl_area=[0, 0, 0, 0, 0, 0, 0]
  z-3 : Outport
  wires:
  ASR/1(dout) -> z-3/1
  " "/1 -> Register4/1
  Register4/1 -> ASR/1(din)
  " reset"/1 -> Register4/2

== system xrbsComm_r3/White Gaussian  Noise Generator/Box-Muller3/fr1/lfsr_17_2/x7 ==
  " " : Inport
  reset : Inport  Port=2
  ASR : Subsystem  mask{init=[init(2) init(1)]}
      mask prompts: init "Initial Value"
      mask init:
      | init_size = size(init);
      | asr_length = init_size(2);
  Register4 : xbsIndex_r3/Register  init=init(3)  reg_only_valid=off  explicit_period=on  period=-1  rst=on  en=off  out_en=off  dbl_ovrd=off
      settings: xl_area=[0, 0, 0, 0, 0, 0, 0]
  z-3 : Outport
  wires:
  " "/1 -> Register4/1
  ASR/1(dout) -> z-3/1
  Register4/1 -> ASR/1(din)
  reset/1 -> Register4/2

== system xrbsComm_r3/White Gaussian  Noise Generator/Box-Muller3/fr1/lfsr_25_2/x1 ==
  " " : Inport
  reset : Inport  Port=2
  ASR : Subsystem  mask{init=[init(4) init(3) init(2) init(1)]}
      mask prompts: init "Initial Value"
      mask init:
      | init_size = size(init);
      | asr_length = init_size(2);
  Register : xbsIndex_r3/Register  init=init(5)  reg_only_valid=off  explicit_period=on  period=-1  rst=on  en=off  out_en=off  dbl_ovrd=off
      settings: xl_area=[0, 0, 0, 0, 0, 0, 0]
  z-5 : Outport
  wires:
  Register/1 -> ASR/1(din)
  ASR/1(dout) -> z-5/1
  " "/1 -> Register/1
  reset/1 -> Register/2

== system xrbsComm_r3/White Gaussian  Noise Generator/Box-Muller3/fr1/lfsr_25_2/x5 ==
  " " : Inport
  reset : Inport  Port=2
  ASR : Subsystem  mask{init=[init(5) init(4) init(3) init(2) init(1)]}
      mask prompts: init "Initial Value"
      mask init:
      | init_size = size(init);
      | asr_length = init_size(2);
  Register : xbsIndex_r3/Register  init=init(6)  reg_only_valid=off  explicit_period=on  period=-1  rst=on  en=off  out_en=off  dbl_ovrd=off
      settings: xl_area=[0, 0, 0, 0, 0, 0, 0]
  z-6 : Outport
  wires:
  Register/1 -> ASR/1(din)
  ASR/1(dout) -> z-6/1
  " "/1 -> Register/1
  reset/1 -> Register/2

== system xrbsComm_r3/White Gaussian  Noise Generator/Box-Muller3/fr1/lfsr_25_2/x6 ==
  " " : Inport
  reset : Inport  Port=2
  ASR : Subsystem  mask{init=[init(4) init(3) init(2) init(1)]}
      mask prompts: init "Initial Value"
      mask init:
      | init_size = size(init);
      | asr_length = init_size(2);
  Register : xbsIndex_r3/Register  init=init(5)  reg_only_valid=off  explicit_period=on  period=-1  rst=on  en=off  out_en=off  dbl_ovrd=off
      settings: xl_area=[0, 0, 0, 0, 0, 0, 0]
  z-5 : Outport
  wires:
  Register/1 -> ASR/1(din)
  ASR/1(dout) -> z-5/1
  " "/1 -> Register/1
  reset/1 -> Register/2

== system xrbsComm_r3/White Gaussian  Noise Generator/Box-Muller3/fr1/lfsr_25_2/x7 ==
  " " : Inport
  reset : Inport  Port=2
  ASR : Subsystem  mask{init=[init(4) init(3) init(2) init(1)]}
      mask prompts: init "Initial Value"
      mask init:
      | init_size = size(init);
      | asr_length = init_size(2);
  Register : xbsIndex_r3/Register  init=init(5)  reg_only_valid=off  explicit_period=on  period=-1  rst=on  en=off  out_en=off  dbl_ovrd=off
      settings: xl_area=[0, 0, 0, 0, 0, 0, 0]
  z-5 : Outport
  wires:
  Register/1 -> ASR/1(din)
  ASR/1(dout) -> z-5/1
  " "/1 -> Register/1
  reset/1 -> Register/2

== system xrbsComm_r3/White Gaussian  Noise Generator/Box-Muller3/fr1/lfsr_29_2/x5 ==
  " " : Inport
  reset : Inport  Port=2
  ASR : Subsystem  mask{init=[init(6) init(5) init(4) init(3) init(2) init(1)]}
      mask prompts: init "Initial Value"
      mask init:
      | init_size = size(init);
      | asr_length = init_size(2);
  Register : xbsIndex_r3/Register  init=init(7)  reg_only_valid=off  explicit_period=on  period=-1  rst=on  en=off  out_en=off  dbl_ovrd=off
      settings: xl_area=[0, 0, 0, 0, 0, 0, 0]
  z-7 : Outport
  wires:
  ASR/1(dout) -> z-7/1
  Register/1 -> ASR/1(din)
  " "/1 -> Register/1
  reset/1 -> Register/2

== system xrbsComm_r3/White Gaussian  Noise Generator/Box-Muller3/fr1/lfsr_29_2/x6 ==
  " " : Inport
  reset : Inport  Port=2
  ASR : Subsystem  mask{init=[init(5) init(4) init(3) init(2) init(1)]}
      mask prompts: init "Initial Value"
      mask init:
      | init_size = size(init);
      | asr_length = init_size(2);
  Register : xbsIndex_r3/Register  init=init(6)  reg_only_valid=off  explicit_period=on  period=-1  rst=on  en=off  out_en=off  dbl_ovrd=off
      settings: xl_area=[0, 0, 0, 0, 0, 0, 0]
  z-6 : Outport
  wires:
  ASR/1(dout) -> z-6/1
  Register/1 -> ASR/1(din)
  " "/1 -> Register/1
  reset/1 -> Register/2

== system xrbsComm_r3/White Gaussian  Noise Generator/Box-Muller3/fr1/lfsr_29_2/x7 ==
  " " : Inport
  reset : Inport  Port=2
  ASR : Subsystem  mask{init=[init(5) init(4) init(3) init(2) init(1)]}
      mask prompts: init "Initial Value"
      mask init:
      | init_size = size(init);
      | asr_length = init_size(2);
  Register : xbsIndex_r3/Register  init=init(6)  reg_only_valid=off  explicit_period=on  period=-1  rst=on  en=off  out_en=off  dbl_ovrd=off
      settings: xl_area=[0, 0, 0, 0, 0, 0, 0]
  z-6 : Outport
  wires:
  ASR/1(dout) -> z-6/1
  Register/1 -> ASR/1(din)
  " "/1 -> Register/1
  reset/1 -> Register/2

== system xrbsComm_r3/White Gaussian  Noise Generator/Box-Muller3/fr1/lfsr_29_2/x8 ==
  " " : Inport
  reset : Inport  Port=2
  ASR : Subsystem  mask{init=[init(5) init(4) init(3) init(2) init(1)]}
      mask prompts: init "Initial Value"
      mask init:
      | init_size = size(init);
      | asr_length = init_size(2);
  Register : xbsIndex_r3/Register  init=init(6)  reg_only_valid=off  explicit_period=on  period=-1  rst=on  en=off  out_en=off  dbl_ovrd=off
      settings: xl_area=[0, 0, 0, 0, 0, 0, 0]
  z-6 : Outport
  wires:
  ASR/1(dout) -> z-6/1
  Register/1 -> ASR/1(din)
  " "/1 -> Register/1
  reset/1 -> Register/2

== system xrbsComm_r3/White Gaussian  Noise Generator/Box-Muller3/fr1/lfsr_31_2/x5 ==
  " " : Inport
  reset : Inport  Port=2
  ASR : Subsystem  mask{init=[init(6) init(5) init(4) init(3) init(2) init(1)]}
      mask prompts: init "Initial Value"
      mask init:
      | init_size = size(init);
      | asr_length = init_size(2);
  Register : xbsIndex_r3/Register  init=init(7)  reg_only_valid=off  explicit_period=on  period=-1  rst=on  en=off  out_en=off  dbl_ovrd=off
      settings: xl_area=[0, 0, 0, 0, 0, 0, 0]
  z-7 : Outport
  wires:
  Register/1 -> ASR/1(din)
  ASR/1(dout) -> z-7/1
  " "/1 -> Register/1
  reset/1 -> Register/2

== system xrbsComm_r3/White Gaussian  Noise Generator/Box-Muller3/fr1/lfsr_31_2/x6 ==
  " " : Inport
  reset : Inport  Port=2
  ASR : Subsystem  mask{init=[init(6) init(5) init(4) init(3) init(2) init(1)]}
      mask prompts: init "Initial Value"
      mask init:
      | init_size = size(init);
      | asr_length = init_size(2);
  Register : xbsIndex_r3/Register  init=init(7)  reg_only_valid=off  explicit_period=on  period=-1  rst=on  en=off  out_en=off  dbl_ovrd=off
      settings: xl_area=[0, 0, 0, 0, 0, 0, 0]
  z-7 : Outport
  wires:
  Register/1 -> ASR/1(din)
  " "/1 -> Register/1
  ASR/1(dout) -> z-7/1
  reset/1 -> Register/2

== system xrbsComm_r3/White Gaussian  Noise Generator/Box-Muller3/fr1/lfsr_31_2/x7 ==
  " " : Inport
  reset : Inport  Port=2
  ASR : Subsystem  mask{init=[init(6) init(5) init(4) init(3) init(2) init(1)]}
      mask prompts: init "Initial Value"
      mask init:
      | init_size = size(init);
      | asr_length = init_size(2);
  Register : xbsIndex_r3/Register  init=init(7)  reg_only_valid=off  explicit_period=on  period=-1  rst=on  en=off  out_en=off  dbl_ovrd=off
      settings: xl_area=[0, 0, 0, 0, 0, 0, 0]
  z-7 : Outport
  wires:
  Register/1 -> ASR/1(din)
  ASR/1(dout) -> z-7/1
  " "/1 -> Register/1
  reset/1 -> Register/2

== system xrbsComm_r3/White Gaussian  Noise Generator/Box-Muller3/fr1/lfsr_31_2/x8 ==
  " " : Inport
  reset : Inport  Port=2
  ASR : Subsystem  mask{init=[init(5) init(4) init(3) init(2) init(1)]}
      mask prompts: init "Initial Value"
      mask init:
      | init_size = size(init);
      | asr_length = init_size(2);
  Register : xbsIndex_r3/Register  init=init(6)  reg_only_valid=off  explicit_period=on  period=-1  rst=on  en=off  out_en=off  dbl_ovrd=off
      settings: xl_area=[0, 0, 0, 0, 0, 0, 0]
  z-6 : Outport
  wires:
  Register/1 -> ASR/1(din)
  " "/1 -> Register/1
  ASR/1(dout) -> z-6/1
  reset/1 -> Register/2

== system xrbsComm_r3/White Gaussian  Noise Generator/Box-Muller3/fr1/lfsr_41_2/x1 ==
  " " : Inport
  reset : Inport  Port=2
  ASR : Subsystem  mask{init=[init(8) init(7) init(6) init(5) init(4) init(3) init(2) init(1)]}
      mask prompts: init "Initial Value"
      mask init:
      | init_size = size(init);
      | asr_length = init_size(2);
  Register1 : xbsIndex_r3/Register  init=init(9)  reg_only_valid=off  explicit_period=on  period=-1  rst=on  en=off  out_en=off  dbl_ovrd=off
      settings: xl_area=[0, 0, 0, 0, 0, 0, 0]
  z-9 : Outport
  wires:
  ASR/1(dout) -> z-9/1
  " "/1 -> Register1/1
  Register1/1 -> ASR/1(din)
  reset/1 -> Register1/2
